simulink model "assignment_6_pd_gravity_comp_2022a"  (R2022a)
settings: Solver=VariableStepAuto  StartTime=0.0  StopTime=10  RelTol=1e-3
values from neighbouring files (symbols this model uses):
  dq0 = [0;0;0]    [assignment_10.m]    (also in assignment_11.m; assignment_12.m; assignment_13.m; assignment_6.m)
  Kd = 100    [assignment_10.m]    (also in assignment_11.m = 1000; assignment_12.m; assignment_6.m = 1000; assignment_7.m = diag(2 * xi .* w))
  Kp = 1000    [assignment_10.m]    (also in assignment_11.m = 10000; assignment_12.m; assignment_6.m; assignment_7.m = diag(w .* w))
  q0 = [0;0;0]    [assignment_10.m]    (also in assignment_11.m; assignment_12.m; assignment_13.m = [0; pi/2; -pi/2]; assignment_6.m)
  q_d = [pi/2; pi/4; -pi/3]    [assignment_6.m]    (also in assignment_9.m = [pi/6; pi/4; -pi/2]; main.m = joints_q_dot(1, 2:end))
settings Model: Creator=acesi  LastModifiedBy=Manu
settings ModelReferenceCC: EnableRefExpFcnMdlSchedulingChecks=off
settings RTWCC: Description=Generic Real-Time Target

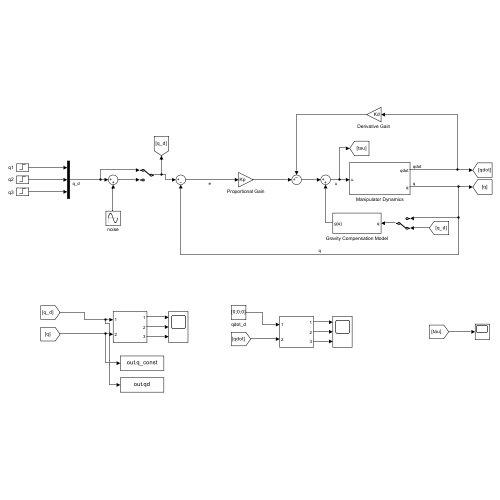
[thumbnail: Simulink's stored preview of the top-level diagram]
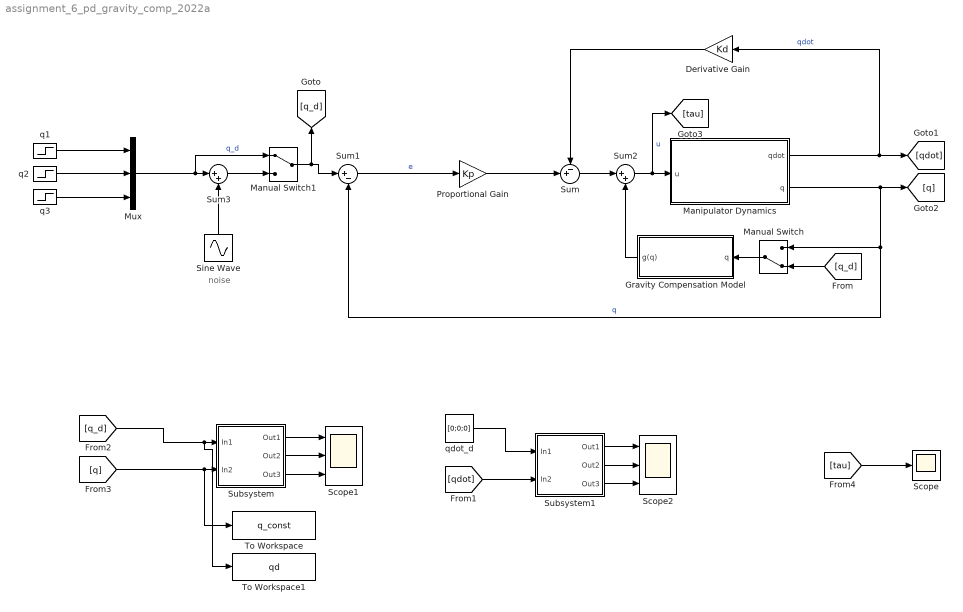
== system assignment_6_pd_gravity_comp_2022a ==
  note: noise
  Derivative Gain : Gain  Gain=Kd
  Gravity Compensation Model : Subsystem
  Manipulator Dynamics : Subsystem
  Manual Switch : ManualSwitch  CurrentSetting=0
  Manual Switch1 : ManualSwitch
  Mux : Mux  Inputs=3
  Proportional Gain : Gain  Gain=Kp
  Scope : Scope
  Scope1 : Scope  NumInputPorts=3
  Scope2 : Scope  NumInputPorts=3
  Sine Wave : Sin  Amplitude=0.05  Frequency=30  SampleTime=0
  Subsystem : Subsystem
  Subsystem1 : Subsystem
  Sum : Sum  Inputs=-+|
  Sum1 : Sum  Inputs=|+-
  Sum2 : Sum  Inputs=|++
  Sum3 : Sum  Inputs=|++
  To Workspace : ToWorkspace  VariableName=q_const  SaveFormat=Timeseries  SampleTime=-1
  To Workspace1 : ToWorkspace  VariableName=qd  SaveFormat=Timeseries  SampleTime=-1
  q1 : Step  After=q_d(1,1)  SampleTime=0
  q2 : Step  After=q_d(2,1)  SampleTime=0
  q3 : Step  After=q_d(3,1)  SampleTime=0
  qdot_d : Constant  Value=[0;0;0]
  wires:
  Proportional Gain/1 -> Sum/2
  Sum1/1 -> Proportional Gain/1  "e"
  Derivative Gain/1 -> Sum/1
  Manipulator Dynamics/1(qdot) -> [qdot], Derivative Gain/1  "qdot"
  Manipulator Dynamics/2(q) -> [q], Manual Switch/1, Sum1/2  "q"
  Sum/1 -> Sum2/1
  Sum2/1 -> Manipulator Dynamics/1(u), [tau]  "u"
  Gravity Compensation Model/1(g(q)) -> Sum2/2
  Mux/1 -> Manual Switch1/1, Sum3/1  "q_d"
  q1/1 -> Mux/1
  q3/1 -> Mux/3
  q2/1 -> Mux/2
  Manual Switch/1 -> Gravity Compensation Model/1(q)
  [q_d] -> Manual Switch/2
  [q_d] -> To Workspace1/1, Subsystem/1(In1)
  [q] -> To Workspace/1, Subsystem/2(In2)
  Subsystem/1(Out1) -> Scope1/1
  Subsystem/2(Out2) -> Scope1/2
  Subsystem/3(Out3) -> Scope1/3
  qdot_d/1 -> Subsystem1/1(In1)
  [qdot] -> Subsystem1/2(In2)
  Subsystem1/1(Out1) -> Scope2/1
  Subsystem1/2(Out2) -> Scope2/2
  Subsystem1/3(Out3) -> Scope2/3
  Sine Wave/1 -> Sum3/2
  Sum3/1 -> Manual Switch1/2
  Manual Switch1/1 -> [q_d], Sum1/1
  [tau] -> Scope/1

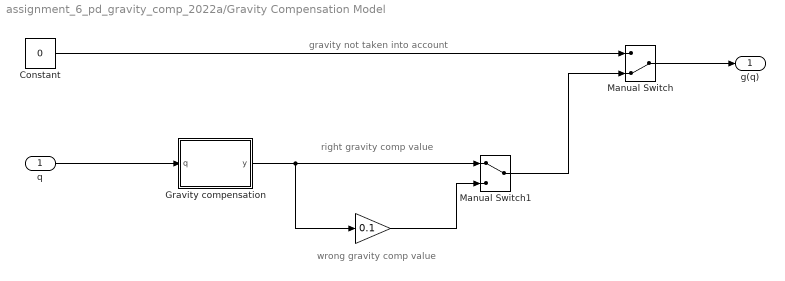
== system assignment_6_pd_gravity_comp_2022a/Gravity Compensation Model ==
  note: wrong gravity comp value
  note: right gravity comp value
  note: gravity not taken into account
  q : Inport
  " " : Gain  Gain=0.1
  Constant : Constant  Value=0
  Gravity compensation : MATLAB Function  TreatAsAtomicUnit=on
  Manual Switch : ManualSwitch  CurrentSetting=0
  Manual Switch1 : ManualSwitch
  g(q) : Outport
  wires:
  Constant/1 -> Manual Switch/1
  Manual Switch/1 -> g(q)/1
  Gravity compensation/1(y) -> " "/1, Manual Switch1/1
  Manual Switch1/1 -> Manual Switch/2
  " "/1 -> Manual Switch1/2
  q/1 -> Gravity compensation/1(q)

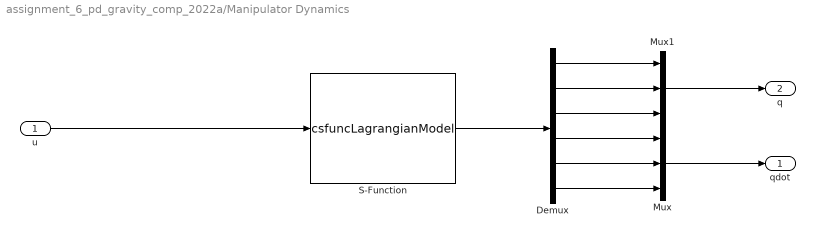
== system assignment_6_pd_gravity_comp_2022a/Manipulator Dynamics ==
  u : Inport
  Demux : Demux  Outputs=6
  Mux : Mux  Inputs=3
  Mux1 : Mux  Inputs=3
  S-Function : S-Function  FunctionName=csfuncLagrangianModel  Parameters=q0 dq0  SFunctionDeploymentMode=off  EnableBusSupport=off
  qdot : Outport
  q : Outport  Port=2
  wires:
  u/1 -> S-Function/1
  S-Function/1 -> Demux/1
  Mux1/1 -> q/1
  Mux/1 -> qdot/1
  Demux/6 -> Mux/3
  Demux/5 -> Mux/2
  Demux/4 -> Mux/1
  Demux/3 -> Mux1/3
  Demux/2 -> Mux1/2
  Demux/1 -> Mux1/1

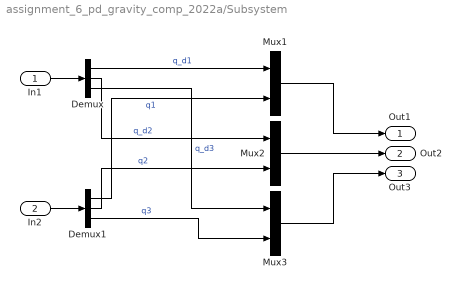
== system assignment_6_pd_gravity_comp_2022a/Subsystem ==
  In1 : Inport
  In2 : Inport  Port=2
  Demux : Demux  Outputs=3
  Demux1 : Demux  Outputs=3
  Mux1 : Mux  Inputs=2
  Mux2 : Mux  Inputs=2
  Mux3 : Mux  Inputs=2
  Out1 : Outport
  Out2 : Outport  Port=2
  Out3 : Outport  Port=3
  wires:
  Demux/1 -> Mux1/1  "q_d1"
  Demux/3 -> Mux3/1  "q_d3"
  Demux/2 -> Mux2/1  "q_d2"
  Demux1/1 -> Mux1/2  "q1"
  Mux2/1 -> Out2/1
  Demux1/3 -> Mux3/2  "q3"
  Demux1/2 -> Mux2/2  "q2"
  Mux3/1 -> Out3/1
  Mux1/1 -> Out1/1
  In2/1 -> Demux1/1
  In1/1 -> Demux/1

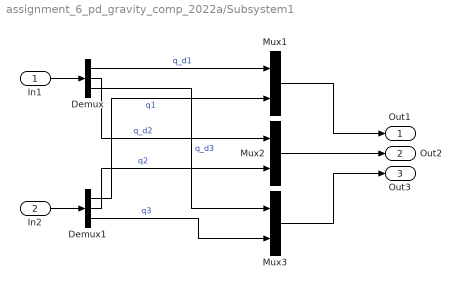
== system assignment_6_pd_gravity_comp_2022a/Subsystem1 ==
  In1 : Inport
  In2 : Inport  Port=2
  Demux : Demux  Outputs=3
  Demux1 : Demux  Outputs=3
  Mux1 : Mux  Inputs=2
  Mux2 : Mux  Inputs=2
  Mux3 : Mux  Inputs=2
  Out1 : Outport
  Out2 : Outport  Port=2
  Out3 : Outport  Port=3
  wires:
  Demux/1 -> Mux1/1  "q_d1"
  Demux/3 -> Mux3/1  "q_d3"
  Demux/2 -> Mux2/1  "q_d2"
  Demux1/1 -> Mux1/2  "q1"
  Mux2/1 -> Out2/1
  Demux1/3 -> Mux3/2  "q3"
  Demux1/2 -> Mux2/2  "q2"
  Mux3/1 -> Out3/1
  Mux1/1 -> Out1/1
  In2/1 -> Demux1/1
  In1/1 -> Demux/1

== matlab function assignment_6_pd_gravity_comp_2022a/Gravity Compensation Model/Gravity compensation ==
  data: q input; y output
function y = g(q)

    y = get_G_hardcoded(q);

end
